simulink model "P3"  (R2020b)
settings: Solver=VariableStepAuto  StartTime=0.0  StopTime=50.0  RelTol=1e-3
settings Model: Creator=stank  LastModifiedBy=stank

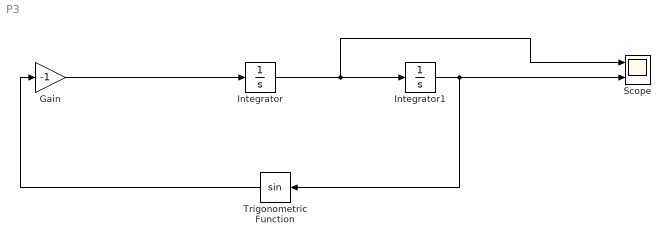
== system P3 ==
  Gain : Gain  Gain=-1
  Integrator : Integrator
  Integrator1 : Integrator  InitialCondition=170/180*pi
  Scope : Scope  NumInputPorts=2
  Trigonometric Function : Trigonometry
  wires:
  Gain/1 -> Integrator/1
  Trigonometric Function/1 -> Gain/1
  Integrator/1 -> Scope/1, Integrator1/1
  Integrator1/1 -> Scope/2, Trigonometric Function/1
